simulink model "Team2_PowerLine_Model_v02"  (R2026a)
settings: Solver=VariableStepAuto  StopTime=2  MaxStep=1e-4
settings Model: Creator=ruyxv  LastModifiedBy=ruyxv

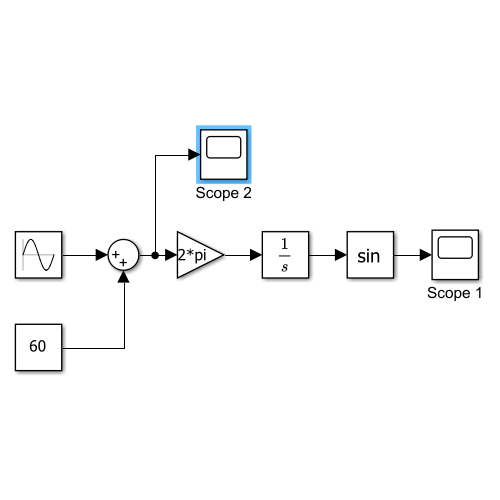
[thumbnail: Simulink's stored preview of the top-level diagram]
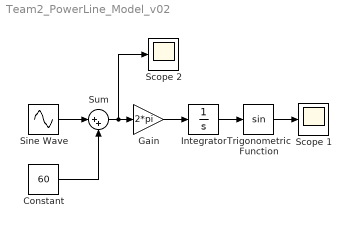
== system Team2_PowerLine_Model_v02 ==
  Constant : Constant  Value=60
  Gain : Gain  Gain=2*pi
  Integrator : Integrator
  Scope 1 : Scope
      settings: ActiveDisplayYMinimum=-1.249999937349582  ActiveDisplayYMaximum=1.2499999534180937
  Scope 2 : Scope
      settings: ActiveDisplayYMinimum=59.975000000035017  ActiveDisplayYMaximum=60.02499999996499
  Sine Wave : Sin  Amplitude=0.02  Frequency=2*pi*0.5  SampleTime=0
  Sum : Sum  Inputs=|++
  Trigonometric Function : Trigonometry
  wires:
  Sine Wave/1 -> Sum/1
  Sum/1 -> Scope 2/1, Gain/1
  Trigonometric Function/1 -> Scope 1/1
  Integrator/1 -> Trigonometric Function/1
  Gain/1 -> Integrator/1
  Constant/1 -> Sum/2
